simulink model "Gun_elev_plant_linear"  (R2022b)
settings: Solver=VariableStepAuto  StartTime=0.0  StopTime=10.0  RelTol=1e-3
undefined symbols (not defined in the file): fix_conseg, JLreg, JMreg, Kkeg, Kveg
settings Model: Creator=ohadformanair  LastModifiedBy=ohadformanair

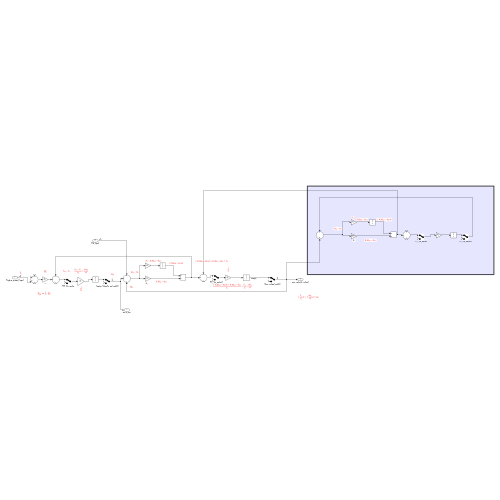
[thumbnail: Simulink's stored preview of the top-level diagram]
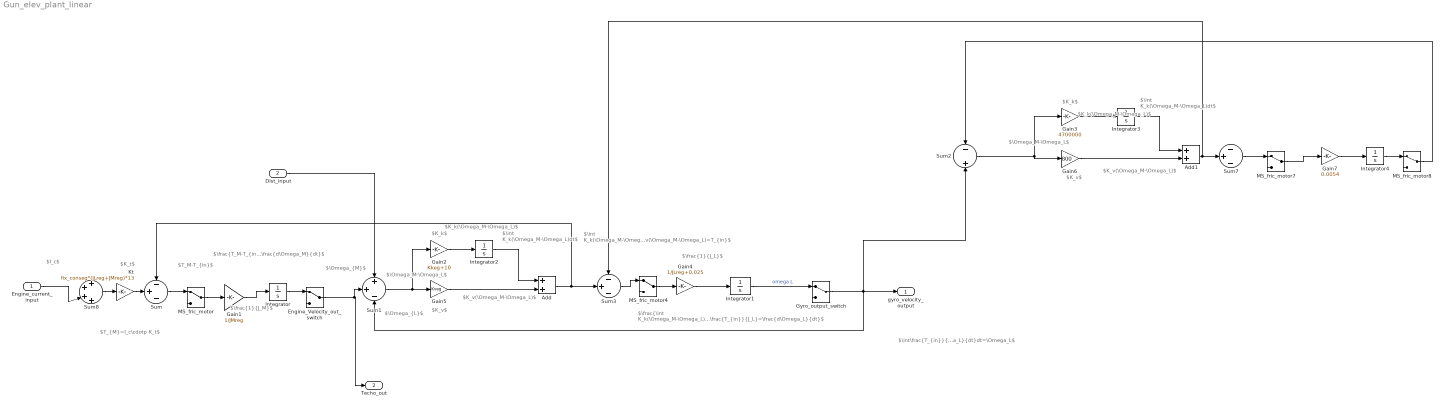
== system Gun_elev_plant_linear ==
  note: $K_v(\Omega_M-\Omega_L)$
  note: $I_c$
  note: $K_k$
  note: $\Omega_{M}$
  note: $\frac{\int K_k(\Omega_M-\Omega_L)dt+K_v(\Omega_M-\Omega_L)}{J_L}=\frac{T_{in}}{J_L}=\frac{d\Omega_L}{dt}$
  note: $K_t$
  note: $\int K_k(\Omega_M-\Omega_L)dt$
  note: $K_v(\Omega_M-\Omega_L)$
  note: $K_v$
  note: $\Omega_M-\Omega_L$
  note: $\int\frac{T_{in}}{J_L}dt=\int\frac{d\Omega_L}{dt}dt=\Omega_L$
  note: $\frac{1}{J_L}$
  note: $K_k$
  note: $\Omega_{L}$
  note: $K_v$
  note: $\frac{1}{J_M}$
  note: $\int K_k(\Omega_M-\Omega_L)dt$
  note: $T_M-T_{in}$
  note: $K_k(\Omega_M-\Omega_L)$
  note: $\frac{T_M-T_{in}}{J_M}=\frac{d\Omega_M}{dt}$
  note: $T_{M}=I_c\cdotp K_t$
  note: $\int K_k(\Omega_M-\Omega_L)dt+K_v(\Omega_M-\Omega_L)=T_{in}$
  note: $\Omega_M-\Omega_L$
  note: $K_k(\Omega_M-\Omega_L)$
  Engine_current_input : Inport
  Dist_input : Inport  Port=2
  Add : Sum
  Add1 : Sum
  Engine_Velocity_out_switch : ManualSwitch
  Gain1 : Gain  Gain=1/JMreg
  Gain2 : Gain  Gain=Kkeg+10
  Gain3 : Gain  Gain=4700000
  Gain4 : Gain  Gain=1/JLreg+0.025
  Gain5 : Gain  Gain=Kveg
  Gain6 : Gain  Gain=800
  Gain7 : Gain  Gain=0.0054
  Gyro_output_switch : ManualSwitch
  Integrator{,1..4} (5 alike) : Integrator
  Kt : Gain  Gain=fix_conseg*(JLreg+JMreg)*13
  MS_fric_motor{,4,7..8} (4 alike) : ManualSwitch
  Sum : Sum  Inputs=-+-
  Sum1 : Sum  Inputs=++-
  Sum2 : Sum  Inputs=-+
  Sum3 : Sum  Inputs=-+-
  Sum7 : Sum  Inputs=-+-
  Sum8 : Sum  Inputs=++++
  gyro_velocity_output : Outport
  Techo_out : Outport  Port=2
  wires:
  MS_fric_motor7/1 -> Gain7/1
  Engine_current_input/1 -> Sum8/3
  Sum2/1 -> Gain6/1, Gain3/1
  Sum8/1 -> Kt/1
  Gain4/1 -> Integrator1/1
  Integrator4/1 -> MS_fric_motor8/1
  Integrator1/1 -> Gyro_output_switch/1  "omega L"
  Gain5/1 -> Add/2
  Integrator2/1 -> Add/1
  Gyro_output_switch/1 -> Sum2/2, Sum1/3, gyro_velocity_output/1
  MS_fric_motor/1 -> Gain1/1
  Sum/1 -> MS_fric_motor/1
  Kt/1 -> Sum/2
  Gain6/1 -> Add1/2
  Gain1/1 -> Integrator/1
  Integrator3/1 -> Add1/1
  Gain7/1 -> Integrator4/1
  Gain3/1 -> Integrator3/1
  Sum1/1 -> Gain5/1, Gain2/1
  Add/1 -> Sum3/2, Sum/1
  Gain2/1 -> Integrator2/1
  Engine_Velocity_out_switch/1 -> Techo_out/1, Sum1/2
  MS_fric_motor8/1 -> Sum2/1
  Sum3/1 -> MS_fric_motor4/1
  Sum7/1 -> MS_fric_motor7/1
  Add1/1 -> Sum7/2, Sum3/1
  MS_fric_motor4/1 -> Gain4/1
  Integrator/1 -> Engine_Velocity_out_switch/1
  Dist_input/1 -> Sum1/1
